simulink model "Model"  (R2024b)
settings: Solver=VariableStepAuto  StartTime=0.0  StopTime=30  MaxStep=0.001  RelTol=1e-4
PostLoadFcn:
  | SIM_setup
values from neighbouring files (symbols this model uses):
  A = 1.1    [RT14e_Parameters.m]    (also in RT15e_Parameters.m = 1.088; RT15evo_Parameters.m = 1.088; SIM_setup.m = 1.12)
  Aero_balance = 55    [RT14e_Parameters.m]    (also in RT15e_Parameters.m; RT15evo_Parameters.m; SIM_setup.m = 0.55)
  air_density = 1.29    [SIM_setup.m]
  Br_coef_of_friction_F = 0.33    [RT14e_Parameters.m]    (also in RT15e_Parameters.m; RT15evo_Parameters.m; SIM_setup.m = 0.25)
  Br_coef_of_friction_R = 0.33    [RT14e_Parameters.m]    (also in RT15e_Parameters.m; RT15evo_Parameters.m; SIM_setup.m = 0.25)
  Br_pistons_area_F = 3617.26/1e6    (= 0.00361726)    [RT14e_Parameters.m]    (also in RT15e_Parameters.m; RT15evo_Parameters.m; SIM_setup.m)
  Br_pistons_area_R = 2026.83/1e6    (= 0.00202683)    [RT14e_Parameters.m]    (also in RT15e_Parameters.m; RT15evo_Parameters.m; SIM_setup.m)
  Cd = 1.387    [SIM_setup.m]
  Cl = 3.299    [SIM_setup.m]
  CoG_z = 0.35    [RT14e_Parameters.m]    (also in RT15e_Parameters.m = 0.28495; RT15evo_Parameters.m = 0.28495; SIM_setup.m = 0.328)
  Default_Fz_F = g*(Mass*(Lr/Wheelbase))    [RT14e_Parameters.m]    (also in RT15e_Parameters.m; RT15evo_Parameters.m; SIM_setup.m = 608.22)
  Default_Fz_R = g*(Mass*(Lf/Wheelbase))    [RT14e_Parameters.m]    (also in RT15e_Parameters.m; RT15evo_Parameters.m; SIM_setup.m = 774.99)
  Effective_br_disk_r_F = 0.0905    [RT14e_Parameters.m]    (also in RT15e_Parameters.m; RT15evo_Parameters.m; SIM_setup.m)
  Effective_br_disk_r_R = 0.0895    [RT14e_Parameters.m]    (also in RT15e_Parameters.m; RT15evo_Parameters.m; SIM_setup.m)
  Fx = Data_Fx(2:end,3:end)    [RT14e_Parameters.m]    (also in RT15e_Parameters.m; RT15evo_Parameters.m; SIM_setup.m = Data_Fx(2:end,2:end))
  Fy = Data_Fy(2:end,3:end)    [RT14e_Parameters.m]    (also in RT15e_Parameters.m; RT15evo_Parameters.m; SIM_setup.m = Data_Fy(2:end,2:end))
  Fz = Data_Fy(2:end,2)    [RT14e_Parameters.m]    (also in RT15e_Parameters.m; RT15evo_Parameters.m; SIM_setup.m = Data_Fy(2:end,1))
  Half_track = 0.6    [SIM_setup.m]
  Iz_wehicle = 120    [RT14e_Parameters.m]    (also in RT15e_Parameters.m; RT15evo_Parameters.m; SIM_setup.m)
  Iz_wheel = 0.15    [RT14e_Parameters.m]    (also in RT15e_Parameters.m; RT15evo_Parameters.m; SIM_setup.m)
  Lateral_load_transfer_distribution = 0.55    [SIM_setup.m]
  Lf = Wheelbase - CoG_x    (= 0.77)    [RT14e_Parameters.m]    (also in RT15e_Parameters.m = 0.7504; RT15evo_Parameters.m = 0.7504; SIM_setup.m)
  Lr = Wheelbase - Lf    (= 0.755)    [RT14e_Parameters.m]    (also in RT15e_Parameters.m = 0.7746; RT15evo_Parameters.m = 0.7746; SIM_setup.m)
  Mass = Vehicle_mass + Driver_mass    (= 290)    [RT14e_Parameters.m]    (also in RT15e_Parameters.m = 265; RT15evo_Parameters.m; SIM_setup.m = 300)
  Max_Torque = 29.1    [SIM_setup.m]
  RB_torque_setting_1 = -2    [RT14e_Parameters.m]    (also in RT15e_Parameters.m; RT15evo_Parameters.m; SIM_setup.m)
  RB_torque_setting_10 = -20    [RT14e_Parameters.m]    (also in RT15e_Parameters.m; RT15evo_Parameters.m; SIM_setup.m)
  RB_torque_setting_2 = -4    [RT14e_Parameters.m]    (also in RT15e_Parameters.m; RT15evo_Parameters.m; SIM_setup.m)
  RB_torque_setting_3 = -6    [RT14e_Parameters.m]    (also in RT15e_Parameters.m; RT15evo_Parameters.m; SIM_setup.m)
  RB_torque_setting_4 = -8    [RT14e_Parameters.m]    (also in RT15e_Parameters.m; RT15evo_Parameters.m; SIM_setup.m)
  RB_torque_setting_5 = -10    [RT14e_Parameters.m]    (also in RT15e_Parameters.m; RT15evo_Parameters.m; SIM_setup.m)
  RB_torque_setting_6 = -12    [RT14e_Parameters.m]    (also in RT15e_Parameters.m; RT15evo_Parameters.m; SIM_setup.m)
  RB_torque_setting_7 = -14    [RT14e_Parameters.m]    (also in RT15e_Parameters.m; RT15evo_Parameters.m; SIM_setup.m)
  RB_torque_setting_8 = -16    [RT14e_Parameters.m]    (also in RT15e_Parameters.m; RT15evo_Parameters.m; SIM_setup.m)
  RB_torque_setting_9 = -18    [RT14e_Parameters.m]    (also in RT15e_Parameters.m; RT15evo_Parameters.m; SIM_setup.m)
  SA = Data_Fy(1,3:end)    [RT14e_Parameters.m]    (also in RT15e_Parameters.m; RT15evo_Parameters.m; SIM_setup.m = Data_Fy(1,2:end))
  SR = Data_Fx(1,3:end)    [RT14e_Parameters.m]    (also in RT15e_Parameters.m; RT15evo_Parameters.m; SIM_setup.m = Data_Fx(1,2:end))
  start_time = 182    [SIM_setup.m]
  start_velocity = Xsens_MTI_670_vel.Value(find(Xsens_MTI_670_vel.Time > start_time, 1)) * 1000 / 3600    [SIM_setup.m]
  Steering_angle_table = [0 9.9 19.9 30.14 40.57 51.05 61.29 70.87 79.38 91.9]    [SIM_setup.m]
  Steering_ratio_table = [3.25 3.24 3.23 3.20 3.16 3.10 3.04 2.97 2.90 2.77]    [SIM_setup.m]
  Tire_radius = 0.203    [RT14e_Parameters.m]    (also in RT15e_Parameters.m; RT15evo_Parameters.m; SIM_setup.m)
  Torque_limit_2 = Motor_maximum_torque*0.2    (= 5.82)    [RT14e_Parameters.m]    (also in RT15e_Parameters.m; RT15evo_Parameters.m; SIM_setup.m)
  Torque_limit_3 = Motor_maximum_torque*0.3    (= 8.73)    [RT14e_Parameters.m]    (also in RT15e_Parameters.m; RT15evo_Parameters.m; SIM_setup.m)
  Torque_limit_4 = Motor_maximum_torque*0.4    (= 11.64)    [RT14e_Parameters.m]    (also in RT15e_Parameters.m; RT15evo_Parameters.m; SIM_setup.m)
  Torque_limit_5 = Motor_maximum_torque*0.5    (= 14.55)    [RT14e_Parameters.m]    (also in RT15e_Parameters.m; RT15evo_Parameters.m; SIM_setup.m)
  Torque_limit_6 = Motor_maximum_torque*0.6    (= 17.46)    [RT14e_Parameters.m]    (also in RT15e_Parameters.m; RT15evo_Parameters.m; SIM_setup.m)
  Torque_limit_7 = Motor_maximum_torque*0.7    (= 20.37)    [RT14e_Parameters.m]    (also in RT15e_Parameters.m; RT15evo_Parameters.m; SIM_setup.m)
  Torque_limit_8 = Motor_maximum_torque*0.8    (= 23.28)    [RT14e_Parameters.m]    (also in RT15e_Parameters.m; RT15evo_Parameters.m; SIM_setup.m)
  Torque_limit_9 = 29.1    [RT14e_Parameters.m]    (also in RT15e_Parameters.m; RT15evo_Parameters.m; SIM_setup.m)
  Torque_limit_max = Motor_maximum_torque    (= 29.1)    [RT14e_Parameters.m]    (also in RT15e_Parameters.m; RT15evo_Parameters.m; SIM_setup.m)
  Torque_limit_min = Motor_maximum_torque*0.1    (= 2.91)    [RT14e_Parameters.m]    (also in RT15e_Parameters.m; RT15evo_Parameters.m; SIM_setup.m)
  Transmission_gear_ratio = 12.9    [SIM_setup.m]
  TV_RB_understeer_gradient_1 = -0.5    [RT14e_Parameters.m]    (also in RT15e_Parameters.m; RT15evo_Parameters.m; SIM_setup.m)
  TV_RB_understeer_gradient_10 = 0.005    [RT14e_Parameters.m]    (also in RT15e_Parameters.m; RT15evo_Parameters.m; SIM_setup.m)
  TV_RB_understeer_gradient_2 = -0.1    [RT14e_Parameters.m]    (also in RT15e_Parameters.m; RT15evo_Parameters.m; SIM_setup.m)
  TV_RB_understeer_gradient_3 = 0.08    [RT14e_Parameters.m]    (also in RT15e_Parameters.m; RT15evo_Parameters.m; SIM_setup.m)
  TV_RB_understeer_gradient_4 = 0.06    [RT14e_Parameters.m]    (also in RT15e_Parameters.m; RT15evo_Parameters.m; SIM_setup.m)
  TV_RB_understeer_gradient_5 = 0.05    [RT14e_Parameters.m]    (also in RT15e_Parameters.m; RT15evo_Parameters.m; SIM_setup.m)
  TV_RB_understeer_gradient_6 = 0.04    [RT14e_Parameters.m]    (also in RT15e_Parameters.m; RT15evo_Parameters.m; SIM_setup.m)
  TV_RB_understeer_gradient_7 = 0.03    [RT14e_Parameters.m]    (also in RT15e_Parameters.m; RT15evo_Parameters.m; SIM_setup.m)
  TV_RB_understeer_gradient_8 = 0.02    [RT14e_Parameters.m]    (also in RT15e_Parameters.m; RT15evo_Parameters.m; SIM_setup.m)
  TV_RB_understeer_gradient_9 = 0.01    [RT14e_Parameters.m]    (also in RT15e_Parameters.m; RT15evo_Parameters.m; SIM_setup.m)
  TV_understeer_gradient_1 = -0.5    [RT14e_Parameters.m]    (also in RT15e_Parameters.m; RT15evo_Parameters.m; SIM_setup.m)
  TV_understeer_gradient_10 = 0.002    [RT14e_Parameters.m]    (also in RT15e_Parameters.m; RT15evo_Parameters.m; SIM_setup.m)
  TV_understeer_gradient_2 = -0.1    [RT14e_Parameters.m]    (also in RT15e_Parameters.m; RT15evo_Parameters.m; SIM_setup.m)
  TV_understeer_gradient_3 = 0.06    [RT14e_Parameters.m]    (also in RT15e_Parameters.m; RT15evo_Parameters.m; SIM_setup.m)
  TV_understeer_gradient_4 = 0.05    [RT14e_Parameters.m]    (also in RT15e_Parameters.m; RT15evo_Parameters.m; SIM_setup.m)
  TV_understeer_gradient_5 = 0.04    [RT14e_Parameters.m]    (also in RT15e_Parameters.m; RT15evo_Parameters.m; SIM_setup.m)
  TV_understeer_gradient_6 = 0.03    [RT14e_Parameters.m]    (also in RT15e_Parameters.m; RT15evo_Parameters.m; SIM_setup.m)
  TV_understeer_gradient_7 = 0.02    [RT14e_Parameters.m]    (also in RT15e_Parameters.m; RT15evo_Parameters.m; SIM_setup.m)
  TV_understeer_gradient_8 = 0.01    [RT14e_Parameters.m]    (also in RT15e_Parameters.m; RT15evo_Parameters.m; SIM_setup.m)
  TV_understeer_gradient_9 = 0.005    [RT14e_Parameters.m]    (also in RT15e_Parameters.m; RT15evo_Parameters.m; SIM_setup.m)
  Wheel_base = 1.525    [SIM_setup.m]
  Wheel_rolling_resistance = 0.055    [RT14e_Parameters.m]    (also in RT15e_Parameters.m; RT15evo_Parameters.m; SIM_setup.m)
undefined symbols (not defined in the file or in its folder): Actual_Torque_Value_RL, Actual_Torque_Value_RR, aero_balance, APPS, Brake_Pressure_Front, Brake_Pressure_Rear, lateral_load_transfer_distribution, Steering_position, tire_radius, wheel_base, Xsens_MTI_670_accX, Xsens_MTI_670_accY, Xsens_MTI_670_gyrZ, Xsens_MTI_670_vel, Xsens_Yaw_Rate__deg_s_
libraries: simulink x20, simulink_extras x7, dspstat3 x4, slpidlib x1, slrealtimeloglib x1
(part 3 of 4)

== system Model/Drivetrain/TV Algorithm/Torque Vectoring/Yaw Rate Calculation ==
  Wheel Angle F [deg] : Inport
  SWS VD Parameter 3 : Inport  Port=2
  SWS VD Setup 15 : Inport  Port=3
  Vehicle Speed [km/h] : Inport  Port=4
  " " : Constant  Value=wheel_base
  Add : Sum
  Divide : Product  Inputs=**/
  Divide1 : Product  Inputs=**
  Square : Math  Operator=square
  Understeer Gradeint Selection : Subsystem
      settings: PortSchema="{\"entries\":[{\"content\":{\"sides\":[{\"content\":{\"connectorIds\":[\"In1\",\"In2\"]},\"type\":\"ConnectorPlacement.EquallySpacedRectSide\",\"uuid\":\"bbee3044-93c1-4f00-ad8f-ae9545aae918\"},{\"content\":{\"connectorIds\":[\"Out1\"],\"side\":\"RIGHT\"},\"type\":\"ConnectorPlacement.EquallySpacedRectSide\",\"uuid\":\"d52ebedb-cc23-4f58-8da8-d3f4b5fce62c\"},{\"content\":{\"connectorIds\":[\"In3\"],\"side\":\"TOP\"},\"type\":\"ConnectorPlacement.EquallySpacedRectSide\",\"uuid\":\"93c9d09d-d680-478a-b9be-fd64b3374c94\"}]},\"type\":\"ConnectorPlacement.EquallySpacedConnector\",\"uuid\":\"e2c6614b-4230-44de-856f-0f9866b3d36c\"}],\"packageUris\":[\"http://schema.mathworks.com/mf0/Connector/R2020b\"],\"version\":\"1.0\"}"
  Desired Yaw Rate TV [deg/s] : Outport
  wires:
  " "/1 -> Add/1
  Divide/1 -> Desired Yaw Rate TV [deg/s]/1  "Desired Yaw Rate TV [deg/s]"
  Square/1 -> Divide1/1
  Understeer Gradeint Selection/1(Understeer Gradient) -> Divide1/2
  Divide1/1 -> Add/2
  Add/1 -> Divide/3
  Wheel Angle F [deg]/1 -> Divide/1
  SWS VD Parameter 3/1 -> Understeer Gradeint Selection/1(SWS VD Parameter 3)
  SWS VD Setup 15/1 -> Understeer Gradeint Selection/2(SWS VD Setup 15)
  Vehicle Speed [km/h]/1 -> Square/1, Understeer Gradeint Selection/3(Vehicle Speed [km/h]), Divide/2

== system Model/Tires /Subsystem1/Slip Angle/Slip Angle FL ==
  Y_Velocity : Inport
  Yaw_Rate : Inport  Port=2
  X_Velocity : Inport  Port=3
  Steering_Angle_FL : Inport  Port=4
  Constant : Constant  Value=Lf
  Constant1 : Constant  Value=Half_track
  Divide : Product  Inputs=*/
  Product : Product
  Product1 : Product
  Subtract : Sum
  Subtract1 : Sum  Inputs=-+
  Subtract2 : Sum  Inputs=+-
  Slip_Angle_FL : Outport
  wires:
  Subtract2/1 -> Slip_Angle_FL/1
  Steering_Angle_FL/1 -> Subtract2/2
  Divide/1 -> Subtract2/1
  Subtract1/1 -> Divide/2
  Subtract/1 -> Divide/1
  X_Velocity/1 -> Subtract1/2
  Y_Velocity/1 -> Subtract/1
  Product/1 -> Subtract/2
  Product1/1 -> Subtract1/1
  Constant1/1 -> Product1/2
  Constant/1 -> Product/1
  Yaw_Rate/1 -> Product/2, Product1/1

== system Model/Tires /Subsystem1/Slip Angle/Slip Angle FR ==
  Y_Velocity : Inport
  Yaw_Rate : Inport  Port=2
  X_Velocity : Inport  Port=3
  Steering_Angle_FR : Inport  Port=4
  Constant : Constant  Value=Lf
  Constant1 : Constant  Value=Half_track
  Divide : Product  Inputs=*/
  Product : Product
  Product1 : Product
  Subtract : Sum
  Subtract1 : Sum
  Subtract2 : Sum  Inputs=+-
  Slip_Angle_FR : Outport
  wires:
  Yaw_Rate/1 -> Product1/1, Product/2
  Constant/1 -> Product/1
  Constant1/1 -> Product1/2
  Product1/1 -> Subtract1/1
  Product/1 -> Subtract/2
  Y_Velocity/1 -> Subtract/1
  X_Velocity/1 -> Subtract1/2
  Subtract/1 -> Divide/1
  Subtract1/1 -> Divide/2
  Divide/1 -> Subtract2/1
  Steering_Angle_FR/1 -> Subtract2/2
  Subtract2/1 -> Slip_Angle_FR/1

== system Model/Tires /Subsystem1/Slip Angle/Slip Angle RL ==
  Y_Velocity : Inport
  Yaw_Rate : Inport  Port=2
  X_Velocity : Inport  Port=3
  Constant : Constant  Value=Lr
  Constant1 : Constant  Value=Half_track
  Divide : Product  Inputs=*/
  Product : Product
  Product1 : Product
  Subtract : Sum  Inputs=+-
  Subtract1 : Sum  Inputs=-+
  Slip_Angle_RL : Outport
  wires:
  Subtract1/1 -> Divide/2
  Subtract/1 -> Divide/1
  X_Velocity/1 -> Subtract1/2
  Y_Velocity/1 -> Subtract/1
  Product/1 -> Subtract/2
  Product1/1 -> Subtract1/1
  Constant1/1 -> Product1/2
  Constant/1 -> Product/1
  Yaw_Rate/1 -> Product/2, Product1/1
  Divide/1 -> Slip_Angle_RL/1

== system Model/Tires /Subsystem1/Slip Angle/Slip Angle RR ==
  Y_Velocity : Inport
  Yaw_Rate : Inport  Port=2
  X_Velocity : Inport  Port=3
  Constant : Constant  Value=Lr
  Constant1 : Constant  Value=Half_track
  Divide : Product  Inputs=*/
  Product : Product
  Product1 : Product
  Subtract : Sum  Inputs=+-
  Subtract1 : Sum
  Slip_Angle_RR : Outport
  wires:
  Yaw_Rate/1 -> Product1/1, Product/2
  Constant/1 -> Product/1
  Constant1/1 -> Product1/2
  Product1/1 -> Subtract1/1
  Product/1 -> Subtract/2
  Y_Velocity/1 -> Subtract/1
  X_Velocity/1 -> Subtract1/2
  Subtract/1 -> Divide/1
  Subtract1/1 -> Divide/2
  Divide/1 -> Slip_Angle_RR/1

== system Model/Tires /Subsystem1/Slip Ratio/Slip ratio FL ==
  Wheel_Angular_Speed_FR [rad/s] : Inport
  X_Velocity [m/s] : Inport  Port=2
  Constant : Constant
  Constant4 : Constant  Value=Tire_radius
  Divide : Product  Inputs=**/
  Subtract : Sum  Inputs=+-
  Slip_Ratio_FL : Outport
  wires:
  Constant4/1 -> Divide/1
  X_Velocity [m/s]/1 -> Divide/3
  Wheel_Angular_Speed_FR [rad/s]/1 -> Divide/2
  Constant/1 -> Subtract/2
  Subtract/1 -> Slip_Ratio_FL/1
  Divide/1 -> Subtract/1  "Tire_Slips"

== system Model/Tires /Subsystem1/Slip Ratio/Slip ratio FR ==
  Wheel_Angular_Speed_FL [rad/s] : Inport
  X_Velocity [m/s] : Inport  Port=2
  Constant : Constant
  Constant4 : Constant  Value=Tire_radius
  Divide : Product  Inputs=**/
  Subtract : Sum  Inputs=+-
  Slip _Ratio_FR : Outport
  wires:
  Divide/1 -> Subtract/1  "Tire_Slips"
  Wheel_Angular_Speed_FL [rad/s]/1 -> Divide/2
  X_Velocity [m/s]/1 -> Divide/3
  Constant4/1 -> Divide/1
  Constant/1 -> Subtract/2
  Subtract/1 -> Slip _Ratio_FR/1

== system Model/Tires /Subsystem1/Slip Ratio/Slip ratio RL ==
  Wheel_Angular_Speed_RL [rad/s] : Inport
  X_Velocity [m/s] : Inport  Port=2
  Constant : Constant
  Constant4 : Constant  Value=Tire_radius
  Divide : Product  Inputs=**/
  Subtract : Sum  Inputs=+-
  Slip_Ratio_RL : Outport
  wires:
  Divide/1 -> Subtract/1  "Tire_Slips"
  Wheel_Angular_Speed_RL [rad/s]/1 -> Divide/2
  X_Velocity [m/s]/1 -> Divide/3
  Constant4/1 -> Divide/1
  Constant/1 -> Subtract/2
  Subtract/1 -> Slip_Ratio_RL/1

== system Model/Tires /Subsystem1/Slip Ratio/Slip ratio RR ==
  Wheel_Angular_Speed_RR [rad/s] : Inport
  X_Velocity [m/s] : Inport  Port=2
  Constant : Constant
  Constant4 : Constant  Value=Tire_radius
  Divide : Product  Inputs=**/
  Subtract : Sum  Inputs=+-
  Slip_Ratio_RR : Outport
  wires:
  Constant4/1 -> Divide/1
  X_Velocity [m/s]/1 -> Divide/3
  Wheel_Angular_Speed_RR [rad/s]/1 -> Divide/2
  Divide/1 -> Subtract/1  "Tire_Slips"
  Constant/1 -> Subtract/2
  Subtract/1 -> Slip_Ratio_RR/1

== system Model/Tires /Subsystem1/wheel_speed/FL_Angular_Speed ==
  Torque : Inport
  Rolling_Resistance : Inport  Port=2
  Fx : Inport  Port=3
  Add1 : Sum  Inputs=---
  Bus Selector : BusSelector  OutputSignals=Brake_Torque [Nm].Front.FL
  Bus Selector1 : BusSelector  OutputSignals=Rolling_Resistance_FL
  Constant4 : Constant  Value=Tire_radius
  Gain1 : Gain  Gain=1/Iz_wheel
  Integrator2 : Integrator
  Product : Product
  Saturation : Saturate  UpperLimit=160  LowerLimit=0
  Wheel_Angular_Speed_FL [rad/s] : Outport
  wires:
  Add1/1 -> Gain1/1
  Gain1/1 -> Integrator2/1
  Fx/1 -> Product/2
  Product/1 -> Add1/1
  Constant4/1 -> Product/1
  Saturation/1 -> Wheel_Angular_Speed_FL [rad/s]/1
  Torque/1 -> Bus Selector/1
  Bus Selector/1 -> Add1/2  "<FL>"
  Integrator2/1 -> Saturation/1
  Rolling_Resistance/1 -> Bus Selector1/1
  Bus Selector1/1 -> Add1/3  "<Rolling_Resistance_FL>"

== system Model/Tires /Subsystem1/wheel_speed/FR_Angular_Speed ==
  Torque : Inport
  Rolling_Resistance : Inport  Port=2
  Fx : Inport  Port=3
  Add1 : Sum  Inputs=---
  Bus Selector : BusSelector  OutputSignals=Brake_Torque [Nm].Front.FR
  Bus Selector1 : BusSelector  OutputSignals=Rolling_Resistance_FR
  Constant4 : Constant  Value=Tire_radius
  Gain1 : Gain  Gain=1/Iz_wheel
  Integrator2 : Integrator
  Product : Product
  Saturation : Saturate  UpperLimit=160  LowerLimit=0
  Wheel_Angular_Speed_FR [rad/s] : Outport
  wires:
  Product/1 -> Add1/1
  Fx/1 -> Product/2
  Gain1/1 -> Integrator2/1
  Add1/1 -> Gain1/1
  Constant4/1 -> Product/1
  Saturation/1 -> Wheel_Angular_Speed_FR [rad/s]/1
  Torque/1 -> Bus Selector/1
  Bus Selector/1 -> Add1/2  "<FR>"
  Integrator2/1 -> Saturation/1
  Rolling_Resistance/1 -> Bus Selector1/1
  Bus Selector1/1 -> Add1/3  "<Rolling_Resistance_FR>"

== system Model/Tires /Subsystem1/wheel_speed/RL_Angular_Speed ==
  Torque : Inport
  Rolling_Resistance : Inport  Port=2
  Fx : Inport  Port=3
  Add1 : Sum  Inputs=---+
  Bus Selector : BusSelector  OutputSignals=Brake_Torque [Nm].Rear.RL,Wheel_Torque_Rear.Left
  Bus Selector1 : BusSelector  OutputSignals=Rolling_Resistance_RL
  Constant4 : Constant  Value=Tire_radius
  Gain1 : Gain  Gain=1/Iz_wheel
  Integrator2 : Integrator
  Product : Product
  Saturation : Saturate  UpperLimit=160  LowerLimit=0
  Wheel_Angular_Speed_RL [rad/s] : Outport
  wires:
  Bus Selector/2 -> Add1/4  "<Left>"
  Integrator2/1 -> Saturation/1
  Bus Selector/1 -> Add1/3  "<RL>"
  Torque/1 -> Bus Selector/1
  Saturation/1 -> Wheel_Angular_Speed_RL [rad/s]/1
  Constant4/1 -> Product/1
  Product/1 -> Add1/1
  Fx/1 -> Product/2
  Gain1/1 -> Integrator2/1
  Add1/1 -> Gain1/1
  Rolling_Resistance/1 -> Bus Selector1/1
  Bus Selector1/1 -> Add1/2  "<Rolling_Resistance_RL>"

== system Model/Tires /Subsystem1/wheel_speed/RR_Angular_Speed ==
  Torque : Inport
  Rolling_Resistance : Inport  Port=2
  Fx : Inport  Port=3
  Add1 : Sum  Inputs=---+
  Bus Selector : BusSelector  OutputSignals=Brake_Torque [Nm].Rear.RR,Wheel_Torque_Rear.Right
  Bus Selector1 : BusSelector  OutputSignals=Rolling_Resistance_RR
  Constant4 : Constant  Value=Tire_radius
  Gain1 : Gain  Gain=1/Iz_wheel
  Integrator2 : Integrator
  Product : Product
  Saturation : Saturate  UpperLimit=160  LowerLimit=0
  Wheel_Angular_Speed_RR [rad/s] : Outport
  wires:
  Bus Selector/2 -> Add1/4  "<Right>"
  Integrator2/1 -> Saturation/1
  Torque/1 -> Bus Selector/1
  Saturation/1 -> Wheel_Angular_Speed_RR [rad/s]/1
  Constant4/1 -> Product/1
  Add1/1 -> Gain1/1
  Gain1/1 -> Integrator2/1
  Fx/1 -> Product/2
  Product/1 -> Add1/1
  Bus Selector1/1 -> Add1/2  "<Rolling_Resistance_RR>"
  Rolling_Resistance/1 -> Bus Selector1/1
  Bus Selector/1 -> Add1/3  "<RR>"

== system Model/Tires /Subsystem1/wheel_speed/Subsystem2 ==
  Fz : Inport
  Bus Selector : BusSelector  OutputSignals=Fz_FL,Fz_FR,Fz_RL,Fz_RR
  Bus Creator : BusCreator  Inputs=4
  Demux : Demux
  Gain : Gain  Gain=Tire_radius
  Gain2 : Gain  Gain=Wheel_rolling_resistance
  Mux : Mux
  Rolling_Resistance : Outport
  wires:
  Fz/1 -> Bus Selector/1
  Bus Selector/1 -> Mux/1  "<Fz_FL>"
  Bus Selector/2 -> Mux/2  "<Fz_FR>"
  Bus Selector/3 -> Mux/3  "<Fz_RL>"
  Bus Selector/4 -> Mux/4  "<Fz_RR>"
  Mux/1 -> Gain/1
  Gain/1 -> Gain2/1
  Demux/1 -> Bus Creator/1  "Rolling_Resistance_FL"
  Demux/2 -> Bus Creator/2  "Rolling_Resistance_FR"
  Demux/3 -> Bus Creator/3  "Rolling_Resistance_RL"
  Demux/4 -> Bus Creator/4  "Rolling_Resistance_RR"
  Bus Creator/1 -> Rolling_Resistance/1  "Rolling_Resistance"
  Gain2/1 -> Demux/1

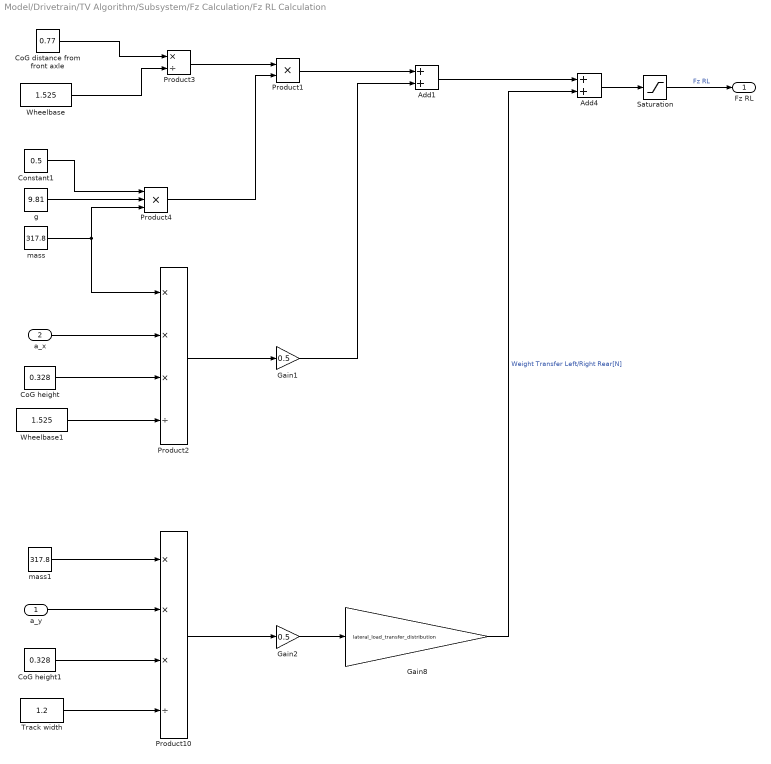
== system Model/Drivetrain/TV Algorithm/Subsystem/Fz Calculation/Fz RL Calculation ==
  a_y : Inport
  a_x : Inport  Port=2
  Add1 : Sum
  Add4 : Sum
  CoG distance from front axle : Constant  Value=0.77
  CoG height : Constant  Value=0.328
  CoG height1 : Constant  Value=0.328
  Constant1 : Constant  Value=0.5
  Gain1 : Gain  Gain=0.5
  Gain2 : Gain  Gain=0.5
  Gain8 : Gain  Gain=lateral_load_transfer_distribution
  Product1 : Product
  Product10 : Product  Inputs=***/
  Product2 : Product  Inputs=***/
  Product3 : Product  Inputs=*/
  Product4 : Product  Inputs=3
  Saturation : Saturate  UpperLimit=10000  LowerLimit=0
  Track width : Constant  Value=1.2
  Wheelbase : Constant  Value=1.525
  Wheelbase1 : Constant  Value=1.525
  g : Constant  Value=9.81
  mass : Constant  Value=317.8
  mass1 : Constant  Value=317.8
  Fz RL : Outport
  wires:
  Wheelbase1/1 -> Product2/4
  Product3/1 -> Product1/1
  CoG distance from front axle/1 -> Product3/1
  Add1/1 -> Add4/1
  Product1/1 -> Add1/1
  g/1 -> Product4/2
  Product4/1 -> Product1/2
  Track width/1 -> Product10/4
  a_y/1 -> Product10/2
  Constant1/1 -> Product4/1
  mass1/1 -> Product10/1
  a_x/1 -> Product2/2
  Wheelbase/1 -> Product3/2
  CoG height/1 -> Product2/3
  CoG height1/1 -> Product10/3
  mass/1 -> Product2/1, Product4/3
  Add4/1 -> Saturation/1
  Saturation/1 -> Fz RL/1  "Fz RL"
  Product2/1 -> Gain1/1
  Product10/1 -> Gain2/1
  Gain1/1 -> Add1/2
  Gain2/1 -> Gain8/1
  Gain8/1 -> Add4/2  "Weight Transfer Left/Right Rear[N]"

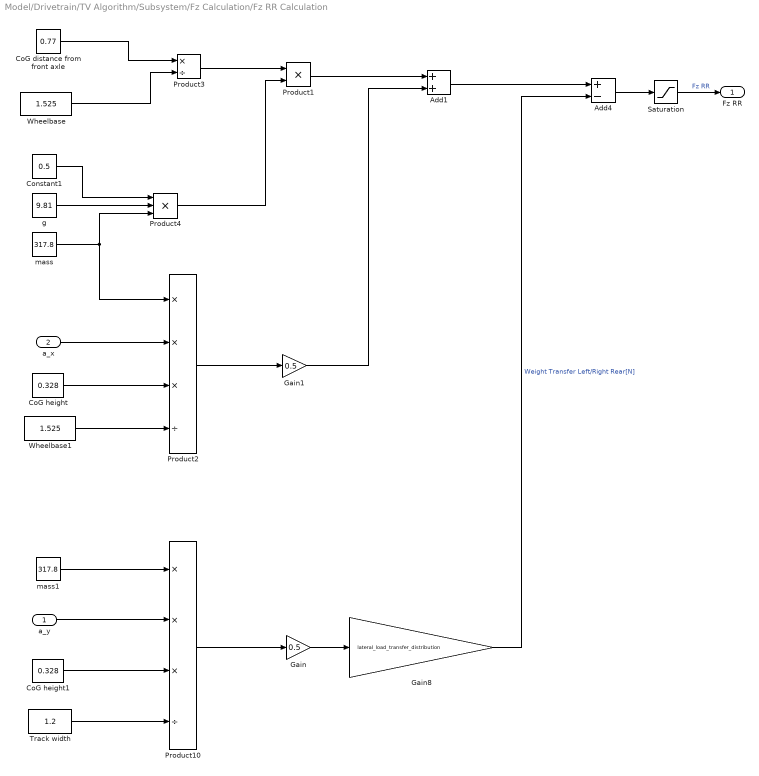
== system Model/Drivetrain/TV Algorithm/Subsystem/Fz Calculation/Fz RR Calculation ==
  a_y : Inport
  a_x : Inport  Port=2
  Add1 : Sum
  Add4 : Sum  Inputs=+-
  CoG distance from front axle : Constant  Value=0.77
  CoG height : Constant  Value=0.328
  CoG height1 : Constant  Value=0.328
  Constant1 : Constant  Value=0.5
  Gain : Gain  Gain=0.5
  Gain1 : Gain  Gain=0.5
  Gain8 : Gain  Gain=lateral_load_transfer_distribution
  Product1 : Product
  Product10 : Product  Inputs=***/
  Product2 : Product  Inputs=***/
  Product3 : Product  Inputs=*/
  Product4 : Product  Inputs=3
  Saturation : Saturate  UpperLimit=10000  LowerLimit=0
  Track width : Constant  Value=1.2
  Wheelbase : Constant  Value=1.525
  Wheelbase1 : Constant  Value=1.525
  g : Constant  Value=9.81
  mass : Constant  Value=317.8
  mass1 : Constant  Value=317.8
  Fz RR : Outport
  wires:
  Product1/1 -> Add1/1
  mass1/1 -> Product10/1
  CoG height1/1 -> Product10/3
  a_y/1 -> Product10/2
  Wheelbase/1 -> Product3/2
  Product4/1 -> Product1/2
  g/1 -> Product4/2
  Track width/1 -> Product10/4
  Constant1/1 -> Product4/1
  mass/1 -> Product2/1, Product4/3
  Add1/1 -> Add4/1
  a_x/1 -> Product2/2
  CoG height/1 -> Product2/3
  Wheelbase1/1 -> Product2/4
  CoG distance from front axle/1 -> Product3/1
  Product3/1 -> Product1/1
  Add4/1 -> Saturation/1
  Saturation/1 -> Fz RR/1  "Fz RR"
  Product10/1 -> Gain/1
  Product2/1 -> Gain1/1
  Gain/1 -> Gain8/1
  Gain1/1 -> Add1/2
  Gain8/1 -> Add4/2  "Weight Transfer Left/Right Rear[N]"

== system Model/Drivetrain/TV Algorithm/Torque Vectoring/RB Yaw Rate Calculation/Understeer Gradeint Selection ==
  SWS VD Parameter 4 : Inport
  Merge1 : Merge  Inputs=11
  Switch Case Action Subsystem11 : Subsystem  TreatAsAtomicUnit=on
  Switch Case Action Subsystem12 : Subsystem  TreatAsAtomicUnit=on
  Switch Case Action Subsystem13 : Subsystem  TreatAsAtomicUnit=on
  Switch Case Action Subsystem14 : Subsystem  TreatAsAtomicUnit=on
  Switch Case Action Subsystem15 : Subsystem  TreatAsAtomicUnit=on
  Switch Case Action Subsystem16 : Subsystem  TreatAsAtomicUnit=on
  Switch Case Action Subsystem17 : Subsystem  TreatAsAtomicUnit=on
  Switch Case Action Subsystem18 : Subsystem  TreatAsAtomicUnit=on
  Switch Case Action Subsystem19 : Subsystem  TreatAsAtomicUnit=on
  Switch Case Action Subsystem20 : Subsystem  TreatAsAtomicUnit=on
  Switch Case Action Subsystem21 : Subsystem  TreatAsAtomicUnit=on
  Switch Case1 : SwitchCase  CaseConditions={1,2,3,4,5,6,7,8,9,10}
  Understeer Gradient : Outport
  wires:
  Merge1/1 -> Understeer Gradient/1
  Switch Case Action Subsystem12/1(Out2) -> Merge1/2
  Switch Case Action Subsystem17/1(Out2) -> Merge1/6
  Switch Case1/7 -> Switch Case Action Subsystem18/Action
  Switch Case Action Subsystem14/1(Out1) -> Merge1/3
  Switch Case1/1 -> Switch Case Action Subsystem11/Action
  Switch Case Action Subsystem11/1(Out1) -> Merge1/1
  Switch Case1/6 -> Switch Case Action Subsystem17/Action
  Switch Case1/4 -> Switch Case Action Subsystem15/Action
  Switch Case1/3 -> Switch Case Action Subsystem14/Action
  Switch Case1/5 -> Switch Case Action Subsystem16/Action
  Switch Case Action Subsystem13/1(Out2) -> Merge1/11
  Switch Case Action Subsystem15/1(Out2) -> Merge1/4
  Switch Case Action Subsystem19/1(Out2) -> Merge1/8
  Switch Case Action Subsystem18/1(Out1) -> Merge1/7
  Switch Case1/8 -> Switch Case Action Subsystem19/Action
  Switch Case Action Subsystem21/1(Out1) -> Merge1/10
  Switch Case Action Subsystem16/1(Out1) -> Merge1/5
  Switch Case Action Subsystem20/1(Out2) -> Merge1/9
  Switch Case1/2 -> Switch Case Action Subsystem12/Action
  Switch Case1/10 -> Switch Case Action Subsystem21/Action
  Switch Case1/9 -> Switch Case Action Subsystem20/Action
  Switch Case1/11 -> Switch Case Action Subsystem13/Action
  SWS VD Parameter 4/1 -> Switch Case1/1

== system Model/Drivetrain/TV Algorithm/Torque Vectoring/Subsystem/Switch Case Action Subsystem ==
  Torque After TV RL [Nm] not saturated : Inport
  Torque After TV RR [Nm] not saturated : Inport  Port=2
  Action Port : ActionPort  ActionPortLabel=case [ 1 ]:
  Bus Creator : BusCreator  Inputs=2
  Saturation : Saturate  UpperLimit=Torque_limit_min  LowerLimit=0
  Saturation1 : Saturate  UpperLimit=Torque_limit_min  LowerLimit=0
  Out1 : Outport
  wires:
  Torque After TV RL [Nm] not saturated/1 -> Saturation/1
  Torque After TV RR [Nm] not saturated/1 -> Saturation1/1
  Saturation/1 -> Bus Creator/1  "Torque After TV RL [Nm]"
  Saturation1/1 -> Bus Creator/2  "Torque After TV RR [Nm]"
  Bus Creator/1 -> Out1/1

== system Model/Drivetrain/TV Algorithm/Torque Vectoring/Subsystem/Switch Case Action Subsystem1 ==
  Torque After TV RL [Nm] not saturated : Inport
  Torque After TV RR [Nm] not saturated : Inport  Port=2
  Action Port : ActionPort  ActionPortLabel=case [ 2 ]:
  Bus Creator : BusCreator  Inputs=2
  Saturation : Saturate  UpperLimit=Torque_limit_2  LowerLimit=0
  Saturation1 : Saturate  UpperLimit=Torque_limit_2  LowerLimit=0
  Out1 : Outport
  wires:
  Saturation1/1 -> Bus Creator/2  "Torque After TV RR [Nm]"
  Torque After TV RR [Nm] not saturated/1 -> Saturation1/1
  Saturation/1 -> Bus Creator/1  "Torque After TV RL [Nm]"
  Bus Creator/1 -> Out1/1
  Torque After TV RL [Nm] not saturated/1 -> Saturation/1

== system Model/Drivetrain/TV Algorithm/Torque Vectoring/Subsystem/Switch Case Action Subsystem10 ==
  Torque After TV RL [Nm] not saturated : Inport
  Torque After TV RR [Nm] not saturated : Inport  Port=2
  Action Port : ActionPort  ActionPortLabel=default:
  Bus Creator : BusCreator  Inputs=2
  Saturation : Saturate  UpperLimit=Torque_limit_max  LowerLimit=0
  Saturation1 : Saturate  UpperLimit=Torque_limit_max  LowerLimit=0
  Out1 : Outport
  wires:
  Saturation1/1 -> Bus Creator/2  "Torque After TV RR [Nm]"
  Torque After TV RR [Nm] not saturated/1 -> Saturation1/1
  Saturation/1 -> Bus Creator/1  "Torque After TV RL [Nm]"
  Bus Creator/1 -> Out1/1
  Torque After TV RL [Nm] not saturated/1 -> Saturation/1

== system Model/Drivetrain/TV Algorithm/Torque Vectoring/Subsystem/Switch Case Action Subsystem2 ==
  Torque After TV RL [Nm] not saturated : Inport
  Torque After TV RR [Nm] not saturated : Inport  Port=2
  Action Port : ActionPort  ActionPortLabel=case [ 3 ]:
  Bus Creator : BusCreator  Inputs=2
  Saturation : Saturate  UpperLimit=Torque_limit_3  LowerLimit=0
  Saturation1 : Saturate  UpperLimit=Torque_limit_3  LowerLimit=0
  Out1 : Outport
  wires:
  Saturation1/1 -> Bus Creator/2  "Torque After TV RR [Nm]"
  Torque After TV RR [Nm] not saturated/1 -> Saturation1/1
  Saturation/1 -> Bus Creator/1  "Torque After TV RL [Nm]"
  Bus Creator/1 -> Out1/1
  Torque After TV RL [Nm] not saturated/1 -> Saturation/1

== system Model/Drivetrain/TV Algorithm/Torque Vectoring/Subsystem/Switch Case Action Subsystem3 ==
  Torque After TV RL [Nm] not saturated : Inport
  Torque After TV RR [Nm] not saturated : Inport  Port=2
  Action Port : ActionPort  ActionPortLabel=case [ 4 ]:
  Bus Creator : BusCreator  Inputs=2
  Saturation : Saturate  UpperLimit=Torque_limit_4  LowerLimit=0
  Saturation1 : Saturate  UpperLimit=Torque_limit_4  LowerLimit=0
  Out1 : Outport
  wires:
  Saturation1/1 -> Bus Creator/2  "Torque After TV RR [Nm]"
  Torque After TV RR [Nm] not saturated/1 -> Saturation1/1
  Saturation/1 -> Bus Creator/1  "Torque After TV RL [Nm]"
  Bus Creator/1 -> Out1/1
  Torque After TV RL [Nm] not saturated/1 -> Saturation/1

== system Model/Drivetrain/TV Algorithm/Torque Vectoring/Subsystem/Switch Case Action Subsystem4 ==
  Torque After TV RL [Nm] not saturated : Inport
  Torque After TV RR [Nm] not saturated : Inport  Port=2
  Action Port : ActionPort  ActionPortLabel=case [ 5 ]:
  Bus Creator : BusCreator  Inputs=2
  Saturation : Saturate  UpperLimit=Torque_limit_5  LowerLimit=0
  Saturation1 : Saturate  UpperLimit=Torque_limit_5  LowerLimit=0
  Out1 : Outport
  wires:
  Saturation1/1 -> Bus Creator/2  "Torque After TV RR [Nm]"
  Torque After TV RR [Nm] not saturated/1 -> Saturation1/1
  Saturation/1 -> Bus Creator/1  "Torque After TV RL [Nm]"
  Bus Creator/1 -> Out1/1
  Torque After TV RL [Nm] not saturated/1 -> Saturation/1

== system Model/Drivetrain/TV Algorithm/Torque Vectoring/Subsystem/Switch Case Action Subsystem5 ==
  Torque After TV RL [Nm] not saturated : Inport
  Torque After TV RR [Nm] not saturated : Inport  Port=2
  Action Port : ActionPort  ActionPortLabel=case [ 6 ]:
  Bus Creator : BusCreator  Inputs=2
  Saturation : Saturate  UpperLimit=Torque_limit_6  LowerLimit=0
  Saturation1 : Saturate  UpperLimit=Torque_limit_6  LowerLimit=0
  Out1 : Outport
  wires:
  Saturation1/1 -> Bus Creator/2  "Torque After TV RR [Nm]"
  Torque After TV RR [Nm] not saturated/1 -> Saturation1/1
  Saturation/1 -> Bus Creator/1  "Torque After TV RL [Nm]"
  Bus Creator/1 -> Out1/1
  Torque After TV RL [Nm] not saturated/1 -> Saturation/1

== system Model/Drivetrain/TV Algorithm/Torque Vectoring/Subsystem/Switch Case Action Subsystem6 ==
  Torque After TV RL [Nm] not saturated : Inport
  Torque After TV RR [Nm] not saturated : Inport  Port=2
  Action Port : ActionPort  ActionPortLabel=case [ 7 ]:
  Bus Creator : BusCreator  Inputs=2
  Saturation : Saturate  UpperLimit=Torque_limit_7  LowerLimit=0
  Saturation1 : Saturate  UpperLimit=Torque_limit_7  LowerLimit=0
  Out1 : Outport
  wires:
  Saturation1/1 -> Bus Creator/2  "Torque After TV RR [Nm]"
  Torque After TV RR [Nm] not saturated/1 -> Saturation1/1
  Saturation/1 -> Bus Creator/1  "Torque After TV RL [Nm]"
  Bus Creator/1 -> Out1/1
  Torque After TV RL [Nm] not saturated/1 -> Saturation/1

== system Model/Drivetrain/TV Algorithm/Torque Vectoring/Subsystem/Switch Case Action Subsystem7 ==
  Torque After TV RL [Nm] not saturated : Inport
  Torque After TV RR [Nm] not saturated : Inport  Port=2
  Action Port : ActionPort  ActionPortLabel=case [ 8 ]:
  Bus Creator : BusCreator  Inputs=2
  Saturation : Saturate  UpperLimit=Torque_limit_8  LowerLimit=0
  Saturation1 : Saturate  UpperLimit=Torque_limit_8  LowerLimit=0
  Out1 : Outport
  wires:
  Saturation1/1 -> Bus Creator/2  "Torque After TV RR [Nm]"
  Torque After TV RR [Nm] not saturated/1 -> Saturation1/1
  Saturation/1 -> Bus Creator/1  "Torque After TV RL [Nm]"
  Bus Creator/1 -> Out1/1
  Torque After TV RL [Nm] not saturated/1 -> Saturation/1

== system Model/Drivetrain/TV Algorithm/Torque Vectoring/Subsystem/Switch Case Action Subsystem8 ==
  Torque After TV RL [Nm] not saturated : Inport
  Torque After TV RR [Nm] not saturated : Inport  Port=2
  Action Port : ActionPort  ActionPortLabel=case [ 9 ]:
  Bus Creator : BusCreator  Inputs=2
  Saturation : Saturate  UpperLimit=Torque_limit_9  LowerLimit=0
  Saturation1 : Saturate  UpperLimit=Torque_limit_9  LowerLimit=0
  Out1 : Outport
  wires:
  Saturation1/1 -> Bus Creator/2  "Torque After TV RR [Nm]"
  Torque After TV RR [Nm] not saturated/1 -> Saturation1/1
  Saturation/1 -> Bus Creator/1  "Torque After TV RL [Nm]"
  Bus Creator/1 -> Out1/1
  Torque After TV RL [Nm] not saturated/1 -> Saturation/1

== system Model/Drivetrain/TV Algorithm/Torque Vectoring/Subsystem/Switch Case Action Subsystem9 ==
  Torque After TV RL [Nm] not saturated : Inport
  Torque After TV RR [Nm] not saturated : Inport  Port=2
  Action Port : ActionPort  ActionPortLabel=case [ 10 ]:
  Bus Creator : BusCreator  Inputs=2
  Saturation : Saturate  UpperLimit=Torque_limit_max  LowerLimit=0
  Saturation1 : Saturate  UpperLimit=Torque_limit_max  LowerLimit=0
  Out1 : Outport
  wires:
  Saturation1/1 -> Bus Creator/2  "Torque After TV RR [Nm]"
  Torque After TV RR [Nm] not saturated/1 -> Saturation1/1
  Saturation/1 -> Bus Creator/1  "Torque After TV RL [Nm]"
  Bus Creator/1 -> Out1/1
  Torque After TV RL [Nm] not saturated/1 -> Saturation/1

== system Model/Drivetrain/TV Algorithm/Torque Vectoring/Subsystem1/Switch Case Action Subsystem ==
  Torque After TV RL [Nm] not saturated : Inport
  Torque After TV RR [Nm] not saturated : Inport  Port=2
  Action Port : ActionPort  ActionPortLabel=case [ 1 ]:
  Bus Creator : BusCreator  Inputs=2
  Saturation : Saturate  UpperLimit=0  LowerLimit=RB_torque_setting_1
  Saturation1 : Saturate  UpperLimit=0  LowerLimit=RB_torque_setting_1
  Out1 : Outport
  wires:
  Bus Creator/1 -> Out1/1
  Saturation1/1 -> Bus Creator/2  "Torque After TV RR [Nm]"
  Saturation/1 -> Bus Creator/1  "Torque After TV RL [Nm]"
  Torque After TV RR [Nm] not saturated/1 -> Saturation1/1
  Torque After TV RL [Nm] not saturated/1 -> Saturation/1

== system Model/Drivetrain/TV Algorithm/Torque Vectoring/Subsystem1/Switch Case Action Subsystem1 ==
  Torque After TV RL [Nm] not saturated : Inport
  Torque After TV RR [Nm] not saturated : Inport  Port=2
  Action Port : ActionPort  ActionPortLabel=case [ 2 ]:
  Bus Creator : BusCreator  Inputs=2
  Saturation : Saturate  UpperLimit=0  LowerLimit=RB_torque_setting_2
  Saturation1 : Saturate  UpperLimit=0  LowerLimit=RB_torque_setting_2
  Out1 : Outport
  wires:
  Torque After TV RL [Nm] not saturated/1 -> Saturation/1
  Bus Creator/1 -> Out1/1
  Saturation/1 -> Bus Creator/1  "Torque After TV RL [Nm]"
  Torque After TV RR [Nm] not saturated/1 -> Saturation1/1
  Saturation1/1 -> Bus Creator/2  "Torque After TV RR [Nm]"

== system Model/Drivetrain/TV Algorithm/Torque Vectoring/Subsystem1/Switch Case Action Subsystem10 ==
  Torque After TV RL [Nm] not saturated : Inport
  Torque After TV RR [Nm] not saturated : Inport  Port=2
  Action Port : ActionPort  ActionPortLabel=default:
  Bus Creator : BusCreator  Inputs=2
  Saturation : Saturate  UpperLimit=Torque_limit_max  LowerLimit=0
  Saturation1 : Saturate  UpperLimit=Torque_limit_max  LowerLimit=0
  Out1 : Outport
  wires:
  Torque After TV RL [Nm] not saturated/1 -> Saturation/1
  Bus Creator/1 -> Out1/1
  Saturation/1 -> Bus Creator/1  "Torque After TV RL [Nm]"
  Torque After TV RR [Nm] not saturated/1 -> Saturation1/1
  Saturation1/1 -> Bus Creator/2  "Torque After TV RR [Nm]"

== system Model/Drivetrain/TV Algorithm/Torque Vectoring/Subsystem1/Switch Case Action Subsystem2 ==
  Torque After TV RL [Nm] not saturated : Inport
  Torque After TV RR [Nm] not saturated : Inport  Port=2
  Action Port : ActionPort  ActionPortLabel=case [ 3 ]:
  Bus Creator : BusCreator  Inputs=2
  Saturation : Saturate  UpperLimit=0  LowerLimit=RB_torque_setting_3
  Saturation1 : Saturate  UpperLimit=0  LowerLimit=RB_torque_setting_3
  Out1 : Outport
  wires:
  Torque After TV RL [Nm] not saturated/1 -> Saturation/1
  Bus Creator/1 -> Out1/1
  Saturation/1 -> Bus Creator/1  "Torque After TV RL [Nm]"
  Torque After TV RR [Nm] not saturated/1 -> Saturation1/1
  Saturation1/1 -> Bus Creator/2  "Torque After TV RR [Nm]"

== system Model/Drivetrain/TV Algorithm/Torque Vectoring/Subsystem1/Switch Case Action Subsystem3 ==
  Torque After TV RL [Nm] not saturated : Inport
  Torque After TV RR [Nm] not saturated : Inport  Port=2
  Action Port : ActionPort  ActionPortLabel=case [ 4 ]:
  Bus Creator : BusCreator  Inputs=2
  Saturation : Saturate  UpperLimit=0  LowerLimit=RB_torque_setting_4
  Saturation1 : Saturate  UpperLimit=0  LowerLimit=RB_torque_setting_4
  Out1 : Outport
  wires:
  Torque After TV RL [Nm] not saturated/1 -> Saturation/1
  Bus Creator/1 -> Out1/1
  Saturation/1 -> Bus Creator/1  "Torque After TV RL [Nm]"
  Torque After TV RR [Nm] not saturated/1 -> Saturation1/1
  Saturation1/1 -> Bus Creator/2  "Torque After TV RR [Nm]"

== system Model/Drivetrain/TV Algorithm/Torque Vectoring/Subsystem1/Switch Case Action Subsystem4 ==
  Torque After TV RL [Nm] not saturated : Inport
  Torque After TV RR [Nm] not saturated : Inport  Port=2
  Action Port : ActionPort  ActionPortLabel=case [ 5 ]:
  Bus Creator : BusCreator  Inputs=2
  Saturation : Saturate  UpperLimit=0  LowerLimit=RB_torque_setting_5
  Saturation1 : Saturate  UpperLimit=0  LowerLimit=RB_torque_setting_5
  Out1 : Outport
  wires:
  Torque After TV RL [Nm] not saturated/1 -> Saturation/1
  Bus Creator/1 -> Out1/1
  Saturation/1 -> Bus Creator/1  "Torque After TV RL [Nm]"
  Torque After TV RR [Nm] not saturated/1 -> Saturation1/1
  Saturation1/1 -> Bus Creator/2  "Torque After TV RR [Nm]"

== system Model/Drivetrain/TV Algorithm/Torque Vectoring/Subsystem1/Switch Case Action Subsystem5 ==
  Torque After TV RL [Nm] not saturated : Inport
  Torque After TV RR [Nm] not saturated : Inport  Port=2
  Action Port : ActionPort  ActionPortLabel=case [ 6 ]:
  Bus Creator : BusCreator  Inputs=2
  Saturation : Saturate  UpperLimit=0  LowerLimit=RB_torque_setting_6
  Saturation1 : Saturate  UpperLimit=0  LowerLimit=RB_torque_setting_6
  Out1 : Outport
  wires:
  Torque After TV RL [Nm] not saturated/1 -> Saturation/1
  Bus Creator/1 -> Out1/1
  Saturation/1 -> Bus Creator/1  "Torque After TV RL [Nm]"
  Torque After TV RR [Nm] not saturated/1 -> Saturation1/1
  Saturation1/1 -> Bus Creator/2  "Torque After TV RR [Nm]"

== system Model/Drivetrain/TV Algorithm/Torque Vectoring/Subsystem1/Switch Case Action Subsystem6 ==
  Torque After TV RL [Nm] not saturated : Inport
  Torque After TV RR [Nm] not saturated : Inport  Port=2
  Action Port : ActionPort  ActionPortLabel=case [ 7 ]:
  Bus Creator : BusCreator  Inputs=2
  Saturation : Saturate  UpperLimit=0  LowerLimit=RB_torque_setting_7
  Saturation1 : Saturate  UpperLimit=0  LowerLimit=RB_torque_setting_7
  Out1 : Outport
  wires:
  Torque After TV RL [Nm] not saturated/1 -> Saturation/1
  Bus Creator/1 -> Out1/1
  Saturation/1 -> Bus Creator/1  "Torque After TV RL [Nm]"
  Torque After TV RR [Nm] not saturated/1 -> Saturation1/1
  Saturation1/1 -> Bus Creator/2  "Torque After TV RR [Nm]"

== system Model/Drivetrain/TV Algorithm/Torque Vectoring/Subsystem1/Switch Case Action Subsystem7 ==
  Torque After TV RL [Nm] not saturated : Inport
  Torque After TV RR [Nm] not saturated : Inport  Port=2
  Action Port : ActionPort  ActionPortLabel=case [ 8 ]:
  Bus Creator : BusCreator  Inputs=2
  Saturation : Saturate  UpperLimit=0  LowerLimit=RB_torque_setting_8
  Saturation1 : Saturate  UpperLimit=0  LowerLimit=RB_torque_setting_8
  Out1 : Outport
  wires:
  Torque After TV RL [Nm] not saturated/1 -> Saturation/1
  Bus Creator/1 -> Out1/1
  Saturation/1 -> Bus Creator/1  "Torque After TV RL [Nm]"
  Torque After TV RR [Nm] not saturated/1 -> Saturation1/1
  Saturation1/1 -> Bus Creator/2  "Torque After TV RR [Nm]"

== system Model/Drivetrain/TV Algorithm/Torque Vectoring/Subsystem1/Switch Case Action Subsystem8 ==
  Torque After TV RL [Nm] not saturated : Inport
  Torque After TV RR [Nm] not saturated : Inport  Port=2
  Action Port : ActionPort  ActionPortLabel=case [ 9 ]:
  Bus Creator : BusCreator  Inputs=2
  Saturation : Saturate  UpperLimit=0  LowerLimit=RB_torque_setting_9
  Saturation1 : Saturate  UpperLimit=0  LowerLimit=RB_torque_setting_9
  Out1 : Outport
  wires:
  Torque After TV RL [Nm] not saturated/1 -> Saturation/1
  Bus Creator/1 -> Out1/1
  Saturation/1 -> Bus Creator/1  "Torque After TV RL [Nm]"
  Torque After TV RR [Nm] not saturated/1 -> Saturation1/1
  Saturation1/1 -> Bus Creator/2  "Torque After TV RR [Nm]"

== system Model/Drivetrain/TV Algorithm/Torque Vectoring/Subsystem1/Switch Case Action Subsystem9 ==
  Torque After TV RL [Nm] not saturated : Inport
  Torque After TV RR [Nm] not saturated : Inport  Port=2
  Action Port : ActionPort  ActionPortLabel=case [ 10 ]:
  Bus Creator : BusCreator  Inputs=2
  Saturation : Saturate  UpperLimit=0  LowerLimit=RB_torque_setting_10
  Saturation1 : Saturate  UpperLimit=0  LowerLimit=RB_torque_setting_10
  Out1 : Outport
  wires:
  Torque After TV RL [Nm] not saturated/1 -> Saturation/1
  Bus Creator/1 -> Out1/1
  Saturation/1 -> Bus Creator/1  "Torque After TV RL [Nm]"
  Torque After TV RR [Nm] not saturated/1 -> Saturation1/1
  Saturation1/1 -> Bus Creator/2  "Torque After TV RR [Nm]"

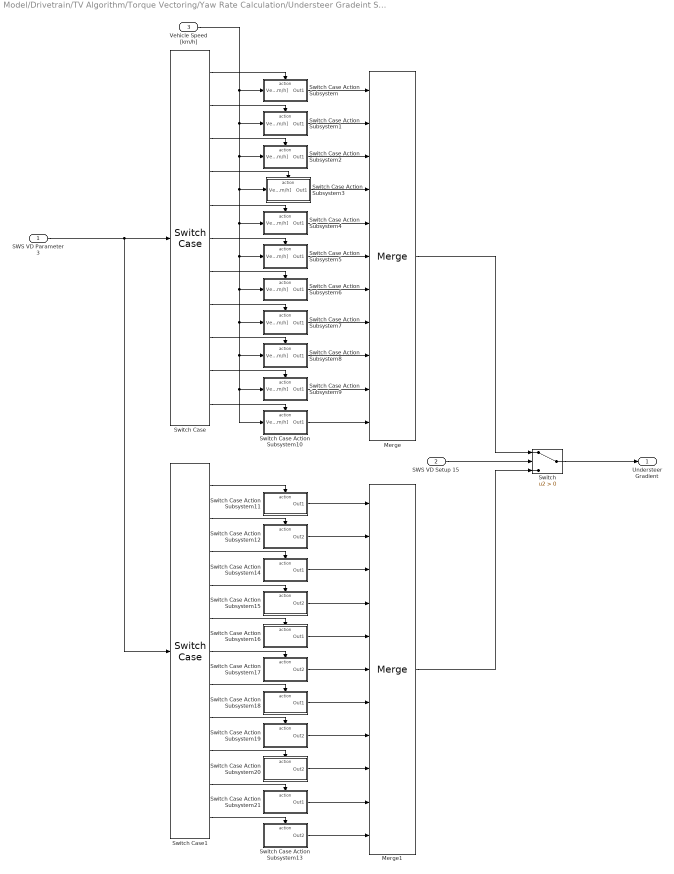
== system Model/Drivetrain/TV Algorithm/Torque Vectoring/Yaw Rate Calculation/Understeer Gradeint Selection ==
  SWS VD Parameter 3 : Inport
  SWS VD Setup 15 : Inport  Port=2
  Vehicle Speed [km/h] : Inport  Port=3
  Merge : Merge  Inputs=11
  Merge1 : Merge  Inputs=11
  Switch : Switch  Criteria=u2 > Threshold  SaturateOnIntegerOverflow=off  InputSameDT=off
  Switch Case : SwitchCase  CaseConditions={1,2,3,4,5,6,7,8,9,10}
  Switch Case Action Subsystem : Subsystem  TreatAsAtomicUnit=on
  Switch Case Action Subsystem1 : Subsystem  TreatAsAtomicUnit=on
  Switch Case Action Subsystem10 : Subsystem  TreatAsAtomicUnit=on
  Switch Case Action Subsystem11 : Subsystem  TreatAsAtomicUnit=on
  Switch Case Action Subsystem12 : Subsystem  TreatAsAtomicUnit=on
  Switch Case Action Subsystem13 : Subsystem  TreatAsAtomicUnit=on
  Switch Case Action Subsystem14 : Subsystem  TreatAsAtomicUnit=on
  Switch Case Action Subsystem15 : Subsystem  TreatAsAtomicUnit=on
  Switch Case Action Subsystem16 : Subsystem  TreatAsAtomicUnit=on
  Switch Case Action Subsystem17 : Subsystem  TreatAsAtomicUnit=on
  Switch Case Action Subsystem18 : Subsystem  TreatAsAtomicUnit=on
  Switch Case Action Subsystem19 : Subsystem  TreatAsAtomicUnit=on
  Switch Case Action Subsystem2 : Subsystem  TreatAsAtomicUnit=on
  Switch Case Action Subsystem20 : Subsystem  TreatAsAtomicUnit=on
  Switch Case Action Subsystem21 : Subsystem  TreatAsAtomicUnit=on
  Switch Case Action Subsystem3 : Subsystem  TreatAsAtomicUnit=on
  Switch Case Action Subsystem4 : Subsystem  TreatAsAtomicUnit=on
  Switch Case Action Subsystem5 : Subsystem  TreatAsAtomicUnit=on
  Switch Case Action Subsystem6 : Subsystem  TreatAsAtomicUnit=on
  Switch Case Action Subsystem7 : Subsystem  TreatAsAtomicUnit=on
  Switch Case Action Subsystem8 : Subsystem  TreatAsAtomicUnit=on
  Switch Case Action Subsystem9 : Subsystem  TreatAsAtomicUnit=on
  Switch Case1 : SwitchCase  CaseConditions={1,2,3,4,5,6,7,8,9,10}
  Understeer Gradient : Outport
  wires:
  Switch Case Action Subsystem1/1(Out1) -> Merge/2
  Switch Case Action Subsystem5/1(Out1) -> Merge/6
  Switch Case/7 -> Switch Case Action Subsystem6/Action
  Switch Case Action Subsystem2/1(Out1) -> Merge/3
  Switch Case/1 -> Switch Case Action Subsystem/Action
  Switch Case Action Subsystem/1(Out1) -> Merge/1
  Switch Case/6 -> Switch Case Action Subsystem5/Action
  Switch Case/4 -> Switch Case Action Subsystem3/Action
  Switch Case/3 -> Switch Case Action Subsystem2/Action
  Switch Case/5 -> Switch Case Action Subsystem4/Action
  Switch Case Action Subsystem10/1(Out1) -> Merge/11
  Switch Case Action Subsystem3/1(Out1) -> Merge/4
  Switch Case Action Subsystem7/1(Out1) -> Merge/8
  Switch Case Action Subsystem6/1(Out1) -> Merge/7
  Switch Case/8 -> Switch Case Action Subsystem7/Action
  Switch Case Action Subsystem9/1(Out1) -> Merge/10
  Switch Case Action Subsystem4/1(Out1) -> Merge/5
  Switch Case Action Subsystem8/1(Out1) -> Merge/9
  Switch Case/2 -> Switch Case Action Subsystem1/Action
  Switch Case/10 -> Switch Case Action Subsystem9/Action
  Switch Case/9 -> Switch Case Action Subsystem8/Action
  Switch Case/11 -> Switch Case Action Subsystem10/Action
  SWS VD Parameter 3/1 -> Switch Case1/1, Switch Case/1
  Switch Case1/11 -> Switch Case Action Subsystem13/Action
  Switch Case1/9 -> Switch Case Action Subsystem20/Action
  Switch Case1/10 -> Switch Case Action Subsystem21/Action
  Switch Case1/2 -> Switch Case Action Subsystem12/Action
  Switch Case Action Subsystem20/1(Out2) -> Merge1/9
  Switch Case Action Subsystem16/1(Out1) -> Merge1/5
  Switch Case Action Subsystem21/1(Out1) -> Merge1/10
  Switch Case1/8 -> Switch Case Action Subsystem19/Action
  Switch Case Action Subsystem18/1(Out1) -> Merge1/7
  Merge1/1 -> Switch/3
  Switch Case Action Subsystem19/1(Out2) -> Merge1/8
  Switch Case Action Subsystem15/1(Out2) -> Merge1/4
  Switch Case Action Subsystem13/1(Out2) -> Merge1/11
  Switch Case1/5 -> Switch Case Action Subsystem16/Action
  Switch Case1/3 -> Switch Case Action Subsystem14/Action
  Switch Case1/4 -> Switch Case Action Subsystem15/Action
  Switch Case1/6 -> Switch Case Action Subsystem17/Action
  Switch Case Action Subsystem11/1(Out1) -> Merge1/1
  Switch Case1/1 -> Switch Case Action Subsystem11/Action
  Switch Case Action Subsystem14/1(Out1) -> Merge1/3
  Switch Case1/7 -> Switch Case Action Subsystem18/Action
  Switch Case Action Subsystem17/1(Out2) -> Merge1/6
  Switch Case Action Subsystem12/1(Out2) -> Merge1/2
  SWS VD Setup 15/1 -> Switch/2
  Merge/1 -> Switch/1
  Switch/1 -> Understeer Gradient/1
  Vehicle Speed [km/h]/1 -> Switch Case Action Subsystem/1(Vehicle Speed [km/h]), Switch Case Action Subsystem1/1(Vehicle Speed [km/h]), Switch Case Action Subsystem2/1(Vehicle Speed [km/h]), Switch Case Action Subsystem3/1(Vehicle Speed [km/h]), Switch Case Action Subsystem4/1(Vehicle Speed [km/h]), Switch Case Action Subsystem5/1(Vehicle Speed [km/h]), Switch Case Action Subsystem6/1(Vehicle Speed [km/h]), Switch Case Action Subsystem7/1(Vehicle Speed [km/h]), Switch Case Action Subsystem8/1(Vehicle Speed [km/h]), Switch Case Action Subsystem10/1(Vehicle Speed [km/h]), Switch Case Action Subsystem9/1(Vehicle Speed [km/h])

== system Model/Drivetrain/TV Algorithm/Torque Vectoring/RB Yaw Rate Calculation/Understeer Gradeint Selection/Switch Case Action Subsystem11 ==
  Action Port : ActionPort  ActionPortLabel=case [ 1 ]:
  Constant1 : Constant  Value=TV_RB_understeer_gradient_1
  Out1 : Outport
  wires:
  Constant1/1 -> Out1/1

== system Model/Drivetrain/TV Algorithm/Torque Vectoring/RB Yaw Rate Calculation/Understeer Gradeint Selection/Switch Case Action Subsystem12 ==
  Action Port : ActionPort  ActionPortLabel=case [ 2 ]:
  Constant : Constant  Value=TV_RB_understeer_gradient_2
  Out2 : Outport
  wires:
  Constant/1 -> Out2/1

== system Model/Drivetrain/TV Algorithm/Torque Vectoring/RB Yaw Rate Calculation/Understeer Gradeint Selection/Switch Case Action Subsystem13 ==
  Action Port : ActionPort  ActionPortLabel=default:
  Constant : Constant  Value=TV_RB_understeer_gradient_6
  Out2 : Outport
  wires:
  Constant/1 -> Out2/1

== system Model/Drivetrain/TV Algorithm/Torque Vectoring/RB Yaw Rate Calculation/Understeer Gradeint Selection/Switch Case Action Subsystem14 ==
  Action Port : ActionPort  ActionPortLabel=case [ 3 ]:
  Constant1 : Constant  Value=TV_RB_understeer_gradient_3
  Out1 : Outport
  wires:
  Constant1/1 -> Out1/1

== system Model/Drivetrain/TV Algorithm/Torque Vectoring/RB Yaw Rate Calculation/Understeer Gradeint Selection/Switch Case Action Subsystem15 ==
  Action Port : ActionPort  ActionPortLabel=case [ 4 ]:
  Constant : Constant  Value=TV_RB_understeer_gradient_4
  Out2 : Outport
  wires:
  Constant/1 -> Out2/1

== system Model/Drivetrain/TV Algorithm/Torque Vectoring/RB Yaw Rate Calculation/Understeer Gradeint Selection/Switch Case Action Subsystem16 ==
  Action Port : ActionPort  ActionPortLabel=case [ 5 ]:
  Constant : Constant  Value=TV_RB_understeer_gradient_5
  Out1 : Outport
  wires:
  Constant/1 -> Out1/1

== system Model/Drivetrain/TV Algorithm/Torque Vectoring/RB Yaw Rate Calculation/Understeer Gradeint Selection/Switch Case Action Subsystem17 ==
  Action Port : ActionPort  ActionPortLabel=case [ 6 ]:
  Constant : Constant  Value=TV_RB_understeer_gradient_6
  Out2 : Outport
  wires:
  Constant/1 -> Out2/1

== system Model/Drivetrain/TV Algorithm/Torque Vectoring/RB Yaw Rate Calculation/Understeer Gradeint Selection/Switch Case Action Subsystem18 ==
  Action Port : ActionPort  ActionPortLabel=case [ 7 ]:
  Constant : Constant  Value=TV_RB_understeer_gradient_7
  Out1 : Outport
  wires:
  Constant/1 -> Out1/1

== system Model/Drivetrain/TV Algorithm/Torque Vectoring/RB Yaw Rate Calculation/Understeer Gradeint Selection/Switch Case Action Subsystem19 ==
  Action Port : ActionPort  ActionPortLabel=case [ 8 ]:
  Constant : Constant  Value=TV_RB_understeer_gradient_8
  Out2 : Outport
  wires:
  Constant/1 -> Out2/1
